simulink model "ParkAssist_Scenario002_cs"  (R2014b)
settings: Solver=ode5  SolverMode=SingleTasking  StartTime=0.0  StopTime=100  FixedStep=1/100  RelTol=1e-3
PreLoadFcn:
  | mbxruntime.callbacks.PreLoadFcn(bdroot);
  | check_NUTS_defined;
  | 
  | assignin('base',['model_closed_' bdroot],false);
  | addpath('../includes_AP');
PostLoadFcn:
  | mbxruntime.callbacks.PostLoadFcn(bdroot);
  | 
  | AP_PlotSpeed;
  | Sim_Stop();
InitFcn:
  | mbxruntime.callbacks.InitFcn(bdroot);
StartFcn:
  | mbxruntime.callbacks.StartFcn(bdroot);
StopFcn:
  | Sim_Stop();
  | 
  | mbxruntime.callbacks.StopFcn(bdroot);
model workspace: external: MAT-File .\ParkAssist_Scenario002_cs_hws.mat (data not in the file)
undefined symbols (not defined in the file or in its folder): mbxruntime, tabledata, warningInitialVelocity, x0
undefined symbols (not defined in the file): ParkAssist_Scenario002_cs_002fddfe84a374e6, ParkAssist_Scenario002_cs_01094a893a7092b9, ParkAssist_Scenario002_cs_02c2e05763b93088, ParkAssist_Scenario002_cs_032149ae54ddfcd1, ParkAssist_Scenario002_cs_03734bce5661314c, ParkAssist_Scenario002_cs_04091ed9282bd749, ParkAssist_Scenario002_cs_068635de1ad515a4, ParkAssist_Scenario002_cs_08968b565ab05e4d, ParkAssist_Scenario002_cs_08eaa26dcd990c9f, ParkAssist_Scenario002_cs_0a721129d3af9f72, ParkAssist_Scenario002_cs_0c5b0314074f54f3, ParkAssist_Scenario002_cs_0e48d515abeb5eec, ParkAssist_Scenario002_cs_1024d8e6ed1cbdcd, ParkAssist_Scenario002_cs_1193d522b107ebab, ParkAssist_Scenario002_cs_11dc16d46c17a7bf, ParkAssist_Scenario002_cs_13631b53806ed88f, ParkAssist_Scenario002_cs_155b57131b5ca1b3, ParkAssist_Scenario002_cs_1a68a29dae7c954c, ParkAssist_Scenario002_cs_1e925263f9fbaeb5, ParkAssist_Scenario002_cs_2102ebaddaee4634, ParkAssist_Scenario002_cs_242d7930853a635b, ParkAssist_Scenario002_cs_26123a651f74a75d, ParkAssist_Scenario002_cs_27077c166553ac4d, ParkAssist_Scenario002_cs_2775446e3f6a532e, ParkAssist_Scenario002_cs_29e1fcc85129d061, ParkAssist_Scenario002_cs_2c6c606bb8eb7e2a, ParkAssist_Scenario002_cs_2f026f6d085d63d4, ParkAssist_Scenario002_cs_2f66cf02f0c1fb02, ParkAssist_Scenario002_cs_2f7abfb8e98983ca, ParkAssist_Scenario002_cs_305144d476c37e1c, ParkAssist_Scenario002_cs_31c4862b0e1d31d2, ParkAssist_Scenario002_cs_3367812933b7aec5, ParkAssist_Scenario002_cs_338ceb4af5dab20a, ParkAssist_Scenario002_cs_359ca59699e4676c, ParkAssist_Scenario002_cs_374ade2de845ad31, ParkAssist_Scenario002_cs_390ab82ad2c54c91, ParkAssist_Scenario002_cs_391805fec31feab6, ParkAssist_Scenario002_cs_3974aed4b8055855, ParkAssist_Scenario002_cs_3a445c73fa984851, ParkAssist_Scenario002_cs_3a54967829cb62c8, ParkAssist_Scenario002_cs_3a60f4e734f7afb5, ParkAssist_Scenario002_cs_3bf2e9c0bde84b70, ParkAssist_Scenario002_cs_3c27f6f01aa99d37, ParkAssist_Scenario002_cs_3cc4b302268f6896, ParkAssist_Scenario002_cs_40419caba47c1546, ParkAssist_Scenario002_cs_42136abd911dac1d, ParkAssist_Scenario002_cs_44b760977392c607, ParkAssist_Scenario002_cs_470135ef0e52cc5f, ParkAssist_Scenario002_cs_48ebb83f5faed864, ParkAssist_Scenario002_cs_4a04bdc7976b10a4, ParkAssist_Scenario002_cs_4b414fc30cdb2355, ParkAssist_Scenario002_cs_4e3c7ad0309ae8ef, ParkAssist_Scenario002_cs_4f1cb442d755f69c, ParkAssist_Scenario002_cs_52f490d0aa621cbf, ParkAssist_Scenario002_cs_53df9d722ee02dea, ParkAssist_Scenario002_cs_5719a2c72af27d7c, ParkAssist_Scenario002_cs_575bfb9c514fb17e, ParkAssist_Scenario002_cs_588d2ca56dde3768, ParkAssist_Scenario002_cs_58ef6c537dd8a6a1, ParkAssist_Scenario002_cs_592f78d63a6470cd ... (+97)
libraries: PreScanUsefulBlocks x57, simulink x55, PreScanSimulinkLibrary x54, simulink_extras x6
(part 9 of 15)

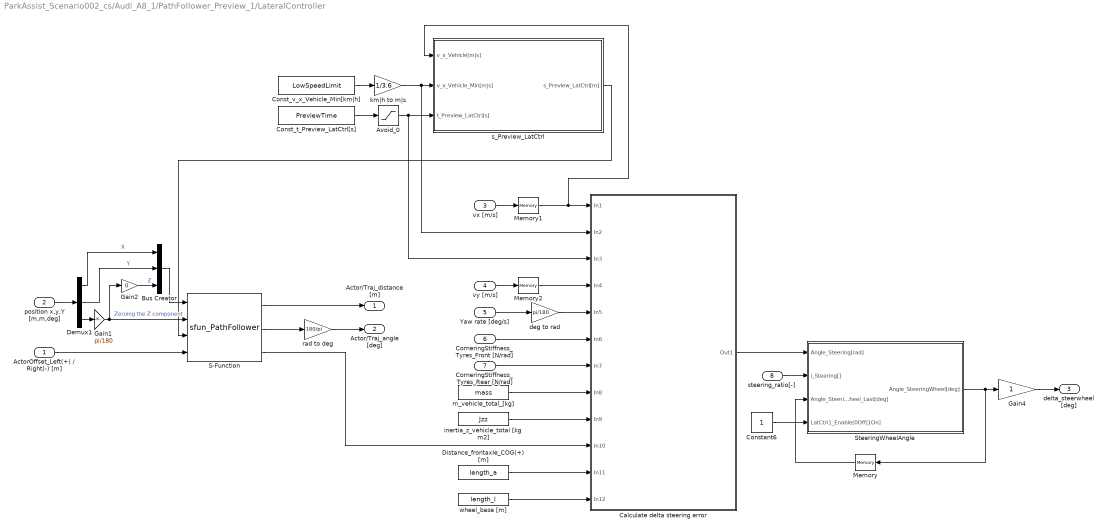
== system ParkAssist_Scenario002_cs/Audi_A8_1/PathFollower_Preview_1/LateralController ==
  ActorOffset_Left(+) / Right(-) [m] : Inport
  position x,y,Y [m,m,deg] : Inport  Port=2
  vx [m/s] : Inport  Port=3
  vy [m/s] : Inport  Port=4
  Yaw rate [deg/s] : Inport  Port=5
  CorneringStiffness_Tyres_Front [N/rad] : Inport  Port=6
  CorneringStiffness_Tyres_Rear [N/rad] : Inport  Port=7
  steering_ratio[-] : Inport  Port=8
  Avoid_0 : Saturate  UpperLimit=1000  LowerLimit=0.1
  Bus Creator : BusCreator  Inputs='X','Y','Z'  OutDataTypeStr=Bus: PRESCAN_XYZ_DATA
  Calculate delta steering error : Subsystem
      mask Display:
      | port_label('input', 1, 'v_x_vehicle [m/s]')
      | port_label('input', 2, 'v_x_vehicle_Min [m/s]')
      | port_label('input', 3, 't_Preview_LatCtrl [s]')
      | port_label('input', 4, 'v_y_vehicle [m/s]')
      | port_label('input', 5, 'yawrate_vehicle [rad/sec]')
      | port_label('input', 6, 'CorneringStiffness_Tyres_Front [N/rad]')
      | port_label('input', 7, 'CorneringStiffness_Tyres_Rear [N/rad]')
      | port_label('input', 8, 'm_vehicle_total [kg]')
      | port_label('input', 9, 'inertia_z_vehicle_total [kg m2]')
      | port_label('input', 10, 'e_Lat [m]')
      | port_label('input', 11, 'Distance_frontaxle_COG(+) [m]')
      | port_label('input', 12, 'wheel_base [m]')
      | port_label('output', 1, 'delta_steeringwheel [rad]')
  Const_t_Preview_LatCtrl[s] : Constant  Value=PreviewTime  SampleTime=CSSampleTime
  Const_v_x_Vehicle_Min[km|h] : Constant  Value=LowSpeedLimit  SampleTime=CSSampleTime
  Constant6 : Constant  SampleTime=CSSampleTime
  Demux1 : Demux  Outputs=3
  Distance_frontaxle_COG(+) [m] : Constant  Value=length_a  SampleTime=CSSampleTime
  Gain1 : Gain  Gain=pi/180
  Gain2 : Gain  Gain=0
  Gain4 : Gain
  Memory : Memory  InheritSampleTime=on
  Memory1 : Memory  InheritSampleTime=on
  Memory2 : Memory  InheritSampleTime=on
  S-Function : S-Function  FunctionName=sfun_PathFollower  Parameters=PathUniqueID,-1  EnableBusSupport=off
  SteeringWheelAngle : Subsystem
  deg to rad : Gain  Gain=pi/180
  inertia_z_vehicle_total [kg m2] : Constant  Value=Jzz  SampleTime=CSSampleTime
  km|h to m|s : Gain  Gain=1/3.6
  m_vehicle_total_[kg] : Constant  Value=mass  SampleTime=CSSampleTime
  rad to deg : Gain  Gain=180/pi
  s_Preview_LatCtrl : Subsystem
  wheel_base [m] : Constant  Value=length_l  SampleTime=CSSampleTime
  Actor/Traj_distance [m] : Outport
  Actor/Traj_angle [deg] : Outport  Port=2
  delta_steerwheel [deg] : Outport  Port=3
  wires:
  Gain2/1 -> Bus Creator/3  "Z"
  Bus Creator/1 -> S-Function/1
  Demux1/2 -> Bus Creator/2  "Y"
  Demux1/1 -> Bus Creator/1  "X"
  s_Preview_LatCtrl/1(s_Preview_LatCtrl[m]) -> S-Function/3
  rad to deg/1 -> Actor/Traj_angle [deg]/1
  km|h to m|s/1 -> Calculate delta steering error/2(In2), s_Preview_LatCtrl/2(v_x_Vehicle_Min[m|s])
  ActorOffset_Left(+) / Right(-) [m]/1 -> S-Function/4
  S-Function/2 -> rad to deg/1
  S-Function/1 -> Actor/Traj_distance [m]/1
  Calculate delta steering error/1(Out1) -> SteeringWheelAngle/1(Angle_Steering[rad])
  vx [m/s]/1 -> Memory1/1
  vy [m/s]/1 -> Memory2/1
  CorneringStiffness_Tyres_Front [N/rad]/1 -> Calculate delta steering error/6(In6)
  m_vehicle_total_[kg]/1 -> Calculate delta steering error/8(In8)
  inertia_z_vehicle_total [kg m2]/1 -> Calculate delta steering error/9(In9)
  steering_ratio[-]/1 -> SteeringWheelAngle/2(i_Steering[])
  SteeringWheelAngle/1(Angle_SteeringWheel[deg]) -> Gain4/1, Memory/1
  Memory/1 -> SteeringWheelAngle/3(Angle_SteeringWheel_Last[deg])
  Constant6/1 -> SteeringWheelAngle/4(LatCtrl1_Enable[0Off|1On])
  Avoid_0/1 -> Calculate delta steering error/3(In3), s_Preview_LatCtrl/3(t_Preview_LatCtrl[s])
  Const_v_x_Vehicle_Min[km|h]/1 -> km|h to m|s/1
  Const_t_Preview_LatCtrl[s]/1 -> Avoid_0/1
  Gain4/1 -> delta_steerwheel [deg]/1
  Distance_frontaxle_COG(+) [m]/1 -> Calculate delta steering error/11(In11)
  CorneringStiffness_Tyres_Rear [N/rad]/1 -> Calculate delta steering error/7(In7)
  Yaw rate [deg/s]/1 -> deg to rad/1
  deg to rad/1 -> Calculate delta steering error/5(In5)
  Gain1/1 -> Gain2/1, S-Function/2  "Zeroing the Z component"
  Demux1/3 -> Gain1/1
  position x,y,Y [m,m,deg]/1 -> Demux1/1
  wheel_base [m]/1 -> Calculate delta steering error/12(In12)
  S-Function/3 -> Calculate delta steering error/10(In10)
  Memory1/1 -> Calculate delta steering error/1(In1), s_Preview_LatCtrl/1(v_x_Vehicle[m|s])
  Memory2/1 -> Calculate delta steering error/4(In4)

== system ParkAssist_Scenario002_cs/Audi_A8_1/PathFollower_Preview_1/LongitudinalController ==
  v_actual [m/s] : Inport
  Desired Velocity [m/s] : Inport  Port=2
  Initial Velocity [m/s] : Inport  Port=3
  Check_Initial_Velocity : Subsystem
  Demux : Demux  Outputs=3
  GearNormal : Constant
  "GearNormal " : Constant
  If Desired Velocity = 0 : Subsystem  TreatAsAtomicUnit=on
  If Desired Velocity ~= 0 : Subsystem  TreatAsAtomicUnit=on
  Memory External IC : Subsystem
  Merge : Merge
  Mux : Mux  Inputs=3
  Mux2 : Mux  Inputs=3
  Sum4 : Sum  Inputs=|+-
  if : If  IfExpression=u1 == 0  SampleTime=CSSampleTime
  throttle [%] : Outport
  brake pressure [bar] : Outport  Port=2
  v0 [m/s] : Outport  Port=3
  Auto_GearShift : Outport  Port=4
  wires:
  v_actual [m/s]/1 -> Check_Initial_Velocity/1(" v_actual_[m|s]"), Memory External IC/1(u)
  Memory External IC/1(y) -> Sum4/2
  Sum4/1 -> If Desired Velocity ~= 0/2(Desired Velocity [m/s])
  Desired Velocity [m/s]/1 -> if/1, Sum4/1
  Initial Velocity [m/s]/1 -> Check_Initial_Velocity/2(Initial_Velocity_[m|s]), Memory External IC/2(IC), v0 [m/s]/1
  GearNormal/1 -> If Desired Velocity = 0/1(In1)
  Merge/1 -> Demux/1
  If Desired Velocity = 0/1(throttle [%]) -> Mux/1
  If Desired Velocity = 0/2(brake pressure [bar]) -> Mux/2
  Mux2/1 -> Merge/2
  Mux/1 -> Merge/1
  Demux/1 -> throttle [%]/1
  Demux/2 -> brake pressure [bar]/1
  Demux/3 -> Auto_GearShift/1
  "GearNormal "/1 -> If Desired Velocity ~= 0/1(In1)
  If Desired Velocity = 0/3(Auto_GearShift) -> Mux/3
  if/2 -> If Desired Velocity ~= 0/Action
  if/1 -> If Desired Velocity = 0/Action
  If Desired Velocity ~= 0/1(throttle [%]) -> Mux2/1
  If Desired Velocity ~= 0/2(brake pressure [bar]) -> Mux2/2
  If Desired Velocity ~= 0/3(Auto_GearShift) -> Mux2/3

== system ParkAssist_Scenario002_cs/Audi_A8_1/SELF_Demux/compas converter ==
  rotz [rad] : Inport
  cart2compas : Subsystem
  rad2deg : Gain  Gain=180/pi
  heading [deg] : Outport
  wires:
  rad2deg/1 -> cart2compas/1(Angle [deg])
  rotz [rad]/1 -> rad2deg/1
  cart2compas/1(heading [deg]) -> heading [deg]/1

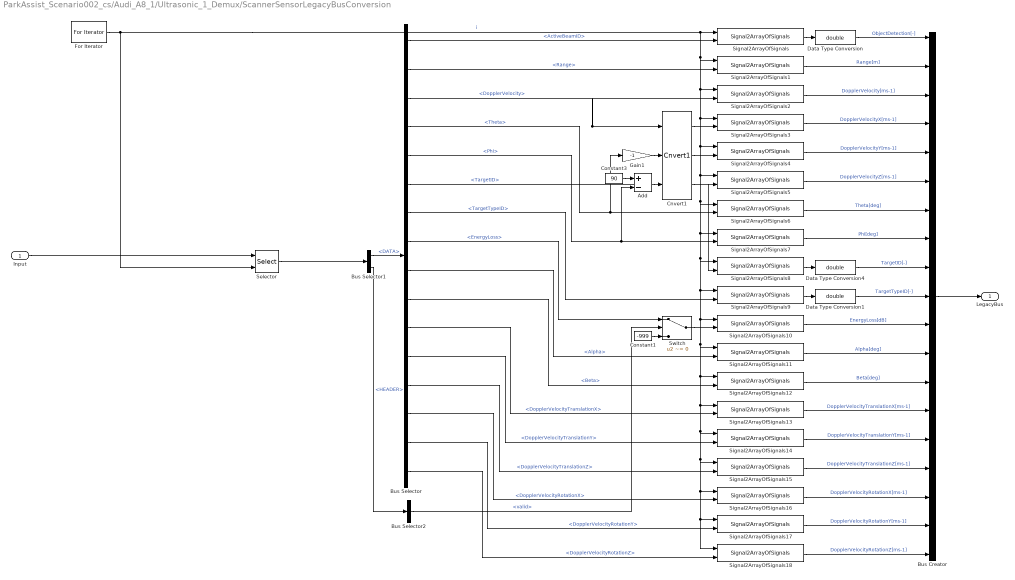
== system ParkAssist_Scenario002_cs/Audi_A8_1/Ultrasonic_1_Demux/ScannerSensorLegacyBusConversion ==
  Input : Inport
  Add : Sum  Inputs=+-
  Bus Creator : BusCreator  Inputs=19
  Bus Selector : BusSelector  OutputSignals=ActiveBeamID,Range,DopplerVelocity,Theta,Phi,TargetID,TargetTypeID,EnergyLoss,Alpha,Beta,DopplerVelocityTranslationX,DopplerVelocityTranslationY,DopplerVelocityTranslationZ,DopplerVelocityRotationX,DopplerVelocityRotationY,DopplerVelocityRotationZ
  Bus Selector1 : BusSelector  OutputSignals=DATA,HEADER
  Bus Selector2 : BusSelector  OutputSignals=valid
  Cnvert1 : PreScanSimulinkLibrary/Cnvert1
  Constant1 : Constant  Value=-999
  Constant3 : Constant  Value=90
  Data Type Conversion : DataTypeConversion  OutDataTypeStr=double  LockScale=on
  Data Type Conversion1 : DataTypeConversion  OutDataTypeStr=double  LockScale=on
  Data Type Conversion4 : DataTypeConversion  OutDataTypeStr=double  LockScale=on
  For Iterator : ForIterator  ResetStates=reset  IterationLimit=MAXMESSAGES
  Gain1 : Gain  Gain=-1
  Selector : Selector  InputPortWidth=MAXMESSAGES  IndexOptions=Index vector (port)  Indices=[1 3]
  Signal2ArrayOfSignals{,1..18} (19 alike) : PreScanUsefulBlocks/Signal2ArrayOfSignals  VECTORLENGTH=MAXMESSAGES
  Switch : Switch  Criteria=u2 ~= 0  Threshold=1
  LegacyBus : Outport
  wires:
  Bus Creator/1 -> LegacyBus/1
  Signal2ArrayOfSignals12/1 -> Bus Creator/13  "Beta[deg]"
  Signal2ArrayOfSignals11/1 -> Bus Creator/12  "Alpha[deg]"
  Signal2ArrayOfSignals10/1 -> Bus Creator/11  "EnergyLoss[dB]"
  Data Type Conversion1/1 -> Bus Creator/10  "TargetTypeID[-]"
  Data Type Conversion4/1 -> Bus Creator/9  "TargetID[-]"
  Signal2ArrayOfSignals7/1 -> Bus Creator/8  "Phi[deg]"
  Signal2ArrayOfSignals6/1 -> Bus Creator/7  "Theta[deg]"
  Signal2ArrayOfSignals5/1 -> Bus Creator/6  "DopplerVelocityZ[ms-1]"
  Signal2ArrayOfSignals4/1 -> Bus Creator/5  "DopplerVelocityY[ms-1]"
  Signal2ArrayOfSignals3/1 -> Bus Creator/4  "DopplerVelocityX[ms-1]"
  Signal2ArrayOfSignals2/1 -> Bus Creator/3  "DopplerVelocity[ms-1]"
  Signal2ArrayOfSignals1/1 -> Bus Creator/2  "Range[m]"
  Data Type Conversion/1 -> Bus Creator/1  "ObjectDetection[-]"
  Signal2ArrayOfSignals9/1 -> Data Type Conversion1/1
  Bus Selector2/1 -> Switch/2  "<valid>"
  Bus Selector1/2 -> Bus Selector2/1  "<HEADER>"
  Bus Selector1/1 -> Bus Selector/1  "<DATA>"
  Switch/1 -> Signal2ArrayOfSignals10/2
  Constant1/1 -> Switch/3
  Bus Selector/8 -> Switch/1  "<EnergyLoss>"
  Selector/1 -> Bus Selector1/1
  Constant3/1 -> Add/1
  Add/1 -> Cnvert1/3
  Gain1/1 -> Cnvert1/2
  Cnvert1/3 -> Signal2ArrayOfSignals5/2
  Cnvert1/2 -> Signal2ArrayOfSignals4/2
  Cnvert1/1 -> Signal2ArrayOfSignals3/2
  Signal2ArrayOfSignals8/1 -> Data Type Conversion4/1
  Bus Selector/1 -> Signal2ArrayOfSignals/2  "<ActiveBeamID>"
  Bus Selector/2 -> Signal2ArrayOfSignals1/2  "<Range>"
  Bus Selector/3 -> Signal2ArrayOfSignals2/2, Cnvert1/1  "<DopplerVelocity>"
  Bus Selector/4 -> Signal2ArrayOfSignals6/2, Gain1/1  "<Theta>"
  Bus Selector/5 -> Signal2ArrayOfSignals7/2, Add/2  "<Phi>"
  Bus Selector/6 -> Signal2ArrayOfSignals8/2  "<TargetID>"
  Bus Selector/7 -> Signal2ArrayOfSignals9/2  "<TargetTypeID>"
  Bus Selector/9 -> Signal2ArrayOfSignals11/2  "<Alpha>"
  Bus Selector/10 -> Signal2ArrayOfSignals12/2  "<Beta>"
  Signal2ArrayOfSignals/1 -> Data Type Conversion/1
  For Iterator/1 -> Signal2ArrayOfSignals11/1, Signal2ArrayOfSignals12/1, Signal2ArrayOfSignals13/1, Signal2ArrayOfSignals14/1, Signal2ArrayOfSignals15/1, Signal2ArrayOfSignals16/1, Signal2ArrayOfSignals17/1, Signal2ArrayOfSignals18/1, Signal2ArrayOfSignals10/1, Signal2ArrayOfSignals9/1, Signal2ArrayOfSignals8/1, Signal2ArrayOfSignals7/1, Signal2ArrayOfSignals6/1, Signal2ArrayOfSignals5/1, Signal2ArrayOfSignals4/1, Signal2ArrayOfSignals3/1, Signal2ArrayOfSignals2/1, Signal2ArrayOfSignals1/1, Signal2ArrayOfSignals/1, Selector/2  "i"
  Input/1 -> Selector/1
  Bus Selector/11 -> Signal2ArrayOfSignals13/2  "<DopplerVelocityTranslationX>"
  Bus Selector/12 -> Signal2ArrayOfSignals14/2  "<DopplerVelocityTranslationY>"
  Bus Selector/13 -> Signal2ArrayOfSignals15/2  "<DopplerVelocityTranslationZ>"
  Bus Selector/14 -> Signal2ArrayOfSignals16/2  "<DopplerVelocityRotationX>"
  Bus Selector/15 -> Signal2ArrayOfSignals17/2  "<DopplerVelocityRotationY>"
  Bus Selector/16 -> Signal2ArrayOfSignals18/2  "<DopplerVelocityRotationZ>"
  Signal2ArrayOfSignals13/1 -> Bus Creator/14  "DopplerVelocityTranslationX[ms-1]"
  Signal2ArrayOfSignals14/1 -> Bus Creator/15  "DopplerVelocityTranslationY[ms-1]"
  Signal2ArrayOfSignals15/1 -> Bus Creator/16  "DopplerVelocityTranslationZ[ms-1]"
  Signal2ArrayOfSignals16/1 -> Bus Creator/17  "DopplerVelocityRotationX[ms-1]"
  Signal2ArrayOfSignals17/1 -> Bus Creator/18  "DopplerVelocityRotationY[ms-1]"
  Signal2ArrayOfSignals18/1 -> Bus Creator/19  "DopplerVelocityRotationZ[ms-1]"

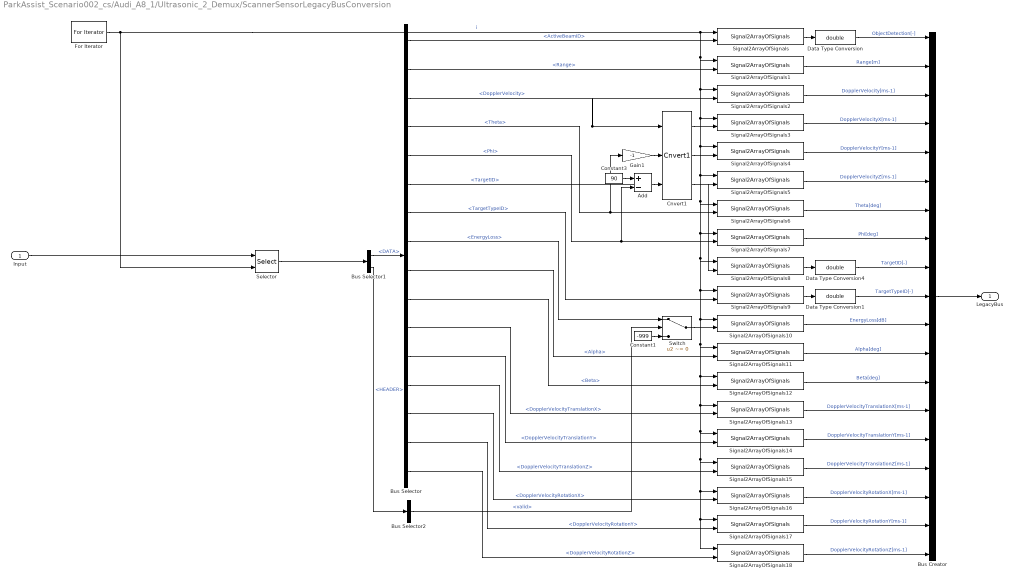
== system ParkAssist_Scenario002_cs/Audi_A8_1/Ultrasonic_2_Demux/ScannerSensorLegacyBusConversion ==
  Input : Inport
  Add : Sum  Inputs=+-
  Bus Creator : BusCreator  Inputs=19
  Bus Selector : BusSelector  OutputSignals=ActiveBeamID,Range,DopplerVelocity,Theta,Phi,TargetID,TargetTypeID,EnergyLoss,Alpha,Beta,DopplerVelocityTranslationX,DopplerVelocityTranslationY,DopplerVelocityTranslationZ,DopplerVelocityRotationX,DopplerVelocityRotationY,DopplerVelocityRotationZ
  Bus Selector1 : BusSelector  OutputSignals=DATA,HEADER
  Bus Selector2 : BusSelector  OutputSignals=valid
  Cnvert1 : PreScanSimulinkLibrary/Cnvert1
  Constant1 : Constant  Value=-999
  Constant3 : Constant  Value=90
  Data Type Conversion : DataTypeConversion  OutDataTypeStr=double  LockScale=on
  Data Type Conversion1 : DataTypeConversion  OutDataTypeStr=double  LockScale=on
  Data Type Conversion4 : DataTypeConversion  OutDataTypeStr=double  LockScale=on
  For Iterator : ForIterator  ResetStates=reset  IterationLimit=MAXMESSAGES
  Gain1 : Gain  Gain=-1
  Selector : Selector  InputPortWidth=MAXMESSAGES  IndexOptions=Index vector (port)  Indices=[1 3]
  Signal2ArrayOfSignals{,1..18} (19 alike) : PreScanUsefulBlocks/Signal2ArrayOfSignals  VECTORLENGTH=MAXMESSAGES
  Switch : Switch  Criteria=u2 ~= 0  Threshold=1
  LegacyBus : Outport
  wires:
  Bus Creator/1 -> LegacyBus/1
  Signal2ArrayOfSignals12/1 -> Bus Creator/13  "Beta[deg]"
  Signal2ArrayOfSignals11/1 -> Bus Creator/12  "Alpha[deg]"
  Signal2ArrayOfSignals10/1 -> Bus Creator/11  "EnergyLoss[dB]"
  Data Type Conversion1/1 -> Bus Creator/10  "TargetTypeID[-]"
  Data Type Conversion4/1 -> Bus Creator/9  "TargetID[-]"
  Signal2ArrayOfSignals7/1 -> Bus Creator/8  "Phi[deg]"
  Signal2ArrayOfSignals6/1 -> Bus Creator/7  "Theta[deg]"
  Signal2ArrayOfSignals5/1 -> Bus Creator/6  "DopplerVelocityZ[ms-1]"
  Signal2ArrayOfSignals4/1 -> Bus Creator/5  "DopplerVelocityY[ms-1]"
  Signal2ArrayOfSignals3/1 -> Bus Creator/4  "DopplerVelocityX[ms-1]"
  Signal2ArrayOfSignals2/1 -> Bus Creator/3  "DopplerVelocity[ms-1]"
  Signal2ArrayOfSignals1/1 -> Bus Creator/2  "Range[m]"
  Data Type Conversion/1 -> Bus Creator/1  "ObjectDetection[-]"
  Signal2ArrayOfSignals9/1 -> Data Type Conversion1/1
  Bus Selector2/1 -> Switch/2  "<valid>"
  Bus Selector1/2 -> Bus Selector2/1  "<HEADER>"
  Bus Selector1/1 -> Bus Selector/1  "<DATA>"
  Switch/1 -> Signal2ArrayOfSignals10/2
  Constant1/1 -> Switch/3
  Bus Selector/8 -> Switch/1  "<EnergyLoss>"
  Selector/1 -> Bus Selector1/1
  Constant3/1 -> Add/1
  Add/1 -> Cnvert1/3
  Gain1/1 -> Cnvert1/2
  Cnvert1/3 -> Signal2ArrayOfSignals5/2
  Cnvert1/2 -> Signal2ArrayOfSignals4/2
  Cnvert1/1 -> Signal2ArrayOfSignals3/2
  Signal2ArrayOfSignals8/1 -> Data Type Conversion4/1
  Bus Selector/1 -> Signal2ArrayOfSignals/2  "<ActiveBeamID>"
  Bus Selector/2 -> Signal2ArrayOfSignals1/2  "<Range>"
  Bus Selector/3 -> Signal2ArrayOfSignals2/2, Cnvert1/1  "<DopplerVelocity>"
  Bus Selector/4 -> Signal2ArrayOfSignals6/2, Gain1/1  "<Theta>"
  Bus Selector/5 -> Signal2ArrayOfSignals7/2, Add/2  "<Phi>"
  Bus Selector/6 -> Signal2ArrayOfSignals8/2  "<TargetID>"
  Bus Selector/7 -> Signal2ArrayOfSignals9/2  "<TargetTypeID>"
  Bus Selector/9 -> Signal2ArrayOfSignals11/2  "<Alpha>"
  Bus Selector/10 -> Signal2ArrayOfSignals12/2  "<Beta>"
  Signal2ArrayOfSignals/1 -> Data Type Conversion/1
  For Iterator/1 -> Signal2ArrayOfSignals11/1, Signal2ArrayOfSignals12/1, Signal2ArrayOfSignals13/1, Signal2ArrayOfSignals14/1, Signal2ArrayOfSignals15/1, Signal2ArrayOfSignals16/1, Signal2ArrayOfSignals17/1, Signal2ArrayOfSignals18/1, Signal2ArrayOfSignals10/1, Signal2ArrayOfSignals9/1, Signal2ArrayOfSignals8/1, Signal2ArrayOfSignals7/1, Signal2ArrayOfSignals6/1, Signal2ArrayOfSignals5/1, Signal2ArrayOfSignals4/1, Signal2ArrayOfSignals3/1, Signal2ArrayOfSignals2/1, Signal2ArrayOfSignals1/1, Signal2ArrayOfSignals/1, Selector/2  "i"
  Input/1 -> Selector/1
  Bus Selector/11 -> Signal2ArrayOfSignals13/2  "<DopplerVelocityTranslationX>"
  Bus Selector/12 -> Signal2ArrayOfSignals14/2  "<DopplerVelocityTranslationY>"
  Bus Selector/13 -> Signal2ArrayOfSignals15/2  "<DopplerVelocityTranslationZ>"
  Bus Selector/14 -> Signal2ArrayOfSignals16/2  "<DopplerVelocityRotationX>"
  Bus Selector/15 -> Signal2ArrayOfSignals17/2  "<DopplerVelocityRotationY>"
  Bus Selector/16 -> Signal2ArrayOfSignals18/2  "<DopplerVelocityRotationZ>"
  Signal2ArrayOfSignals13/1 -> Bus Creator/14  "DopplerVelocityTranslationX[ms-1]"
  Signal2ArrayOfSignals14/1 -> Bus Creator/15  "DopplerVelocityTranslationY[ms-1]"
  Signal2ArrayOfSignals15/1 -> Bus Creator/16  "DopplerVelocityTranslationZ[ms-1]"
  Signal2ArrayOfSignals16/1 -> Bus Creator/17  "DopplerVelocityRotationX[ms-1]"
  Signal2ArrayOfSignals17/1 -> Bus Creator/18  "DopplerVelocityRotationY[ms-1]"
  Signal2ArrayOfSignals18/1 -> Bus Creator/19  "DopplerVelocityRotationZ[ms-1]"

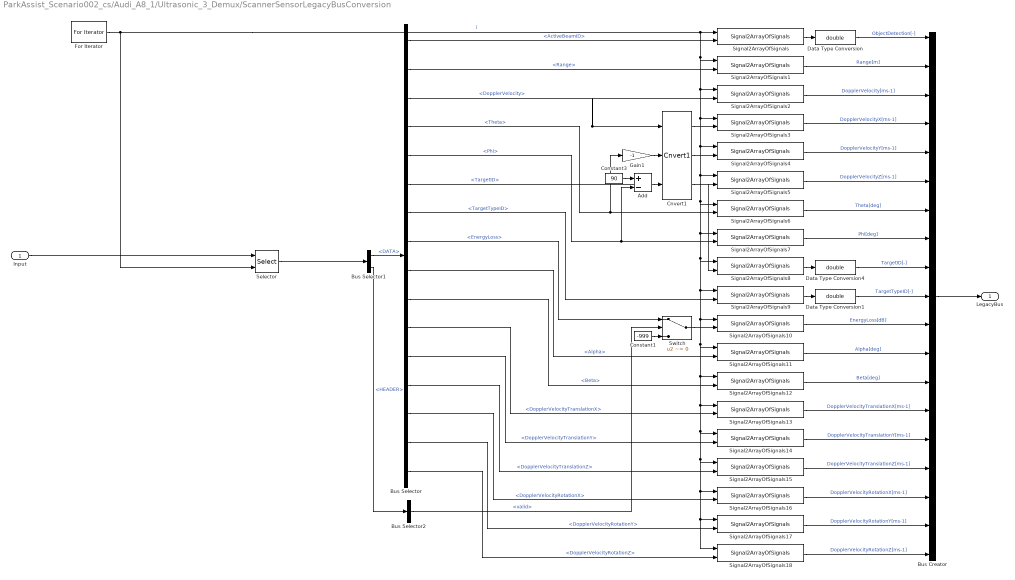
== system ParkAssist_Scenario002_cs/Audi_A8_1/Ultrasonic_3_Demux/ScannerSensorLegacyBusConversion ==
  Input : Inport
  Add : Sum  Inputs=+-
  Bus Creator : BusCreator  Inputs=19
  Bus Selector : BusSelector  OutputSignals=ActiveBeamID,Range,DopplerVelocity,Theta,Phi,TargetID,TargetTypeID,EnergyLoss,Alpha,Beta,DopplerVelocityTranslationX,DopplerVelocityTranslationY,DopplerVelocityTranslationZ,DopplerVelocityRotationX,DopplerVelocityRotationY,DopplerVelocityRotationZ
  Bus Selector1 : BusSelector  OutputSignals=DATA,HEADER
  Bus Selector2 : BusSelector  OutputSignals=valid
  Cnvert1 : PreScanSimulinkLibrary/Cnvert1
  Constant1 : Constant  Value=-999
  Constant3 : Constant  Value=90
  Data Type Conversion : DataTypeConversion  OutDataTypeStr=double  LockScale=on
  Data Type Conversion1 : DataTypeConversion  OutDataTypeStr=double  LockScale=on
  Data Type Conversion4 : DataTypeConversion  OutDataTypeStr=double  LockScale=on
  For Iterator : ForIterator  ResetStates=reset  IterationLimit=MAXMESSAGES
  Gain1 : Gain  Gain=-1
  Selector : Selector  InputPortWidth=MAXMESSAGES  IndexOptions=Index vector (port)  Indices=[1 3]
  Signal2ArrayOfSignals{,1..18} (19 alike) : PreScanUsefulBlocks/Signal2ArrayOfSignals  VECTORLENGTH=MAXMESSAGES
  Switch : Switch  Criteria=u2 ~= 0  Threshold=1
  LegacyBus : Outport
  wires:
  Bus Creator/1 -> LegacyBus/1
  Signal2ArrayOfSignals12/1 -> Bus Creator/13  "Beta[deg]"
  Signal2ArrayOfSignals11/1 -> Bus Creator/12  "Alpha[deg]"
  Signal2ArrayOfSignals10/1 -> Bus Creator/11  "EnergyLoss[dB]"
  Data Type Conversion1/1 -> Bus Creator/10  "TargetTypeID[-]"
  Data Type Conversion4/1 -> Bus Creator/9  "TargetID[-]"
  Signal2ArrayOfSignals7/1 -> Bus Creator/8  "Phi[deg]"
  Signal2ArrayOfSignals6/1 -> Bus Creator/7  "Theta[deg]"
  Signal2ArrayOfSignals5/1 -> Bus Creator/6  "DopplerVelocityZ[ms-1]"
  Signal2ArrayOfSignals4/1 -> Bus Creator/5  "DopplerVelocityY[ms-1]"
  Signal2ArrayOfSignals3/1 -> Bus Creator/4  "DopplerVelocityX[ms-1]"
  Signal2ArrayOfSignals2/1 -> Bus Creator/3  "DopplerVelocity[ms-1]"
  Signal2ArrayOfSignals1/1 -> Bus Creator/2  "Range[m]"
  Data Type Conversion/1 -> Bus Creator/1  "ObjectDetection[-]"
  Signal2ArrayOfSignals9/1 -> Data Type Conversion1/1
  Bus Selector2/1 -> Switch/2  "<valid>"
  Bus Selector1/2 -> Bus Selector2/1  "<HEADER>"
  Bus Selector1/1 -> Bus Selector/1  "<DATA>"
  Switch/1 -> Signal2ArrayOfSignals10/2
  Constant1/1 -> Switch/3
  Bus Selector/8 -> Switch/1  "<EnergyLoss>"
  Selector/1 -> Bus Selector1/1
  Constant3/1 -> Add/1
  Add/1 -> Cnvert1/3
  Gain1/1 -> Cnvert1/2
  Cnvert1/3 -> Signal2ArrayOfSignals5/2
  Cnvert1/2 -> Signal2ArrayOfSignals4/2
  Cnvert1/1 -> Signal2ArrayOfSignals3/2
  Signal2ArrayOfSignals8/1 -> Data Type Conversion4/1
  Bus Selector/1 -> Signal2ArrayOfSignals/2  "<ActiveBeamID>"
  Bus Selector/2 -> Signal2ArrayOfSignals1/2  "<Range>"
  Bus Selector/3 -> Signal2ArrayOfSignals2/2, Cnvert1/1  "<DopplerVelocity>"
  Bus Selector/4 -> Signal2ArrayOfSignals6/2, Gain1/1  "<Theta>"
  Bus Selector/5 -> Signal2ArrayOfSignals7/2, Add/2  "<Phi>"
  Bus Selector/6 -> Signal2ArrayOfSignals8/2  "<TargetID>"
  Bus Selector/7 -> Signal2ArrayOfSignals9/2  "<TargetTypeID>"
  Bus Selector/9 -> Signal2ArrayOfSignals11/2  "<Alpha>"
  Bus Selector/10 -> Signal2ArrayOfSignals12/2  "<Beta>"
  Signal2ArrayOfSignals/1 -> Data Type Conversion/1
  For Iterator/1 -> Signal2ArrayOfSignals11/1, Signal2ArrayOfSignals12/1, Signal2ArrayOfSignals13/1, Signal2ArrayOfSignals14/1, Signal2ArrayOfSignals15/1, Signal2ArrayOfSignals16/1, Signal2ArrayOfSignals17/1, Signal2ArrayOfSignals18/1, Signal2ArrayOfSignals10/1, Signal2ArrayOfSignals9/1, Signal2ArrayOfSignals8/1, Signal2ArrayOfSignals7/1, Signal2ArrayOfSignals6/1, Signal2ArrayOfSignals5/1, Signal2ArrayOfSignals4/1, Signal2ArrayOfSignals3/1, Signal2ArrayOfSignals2/1, Signal2ArrayOfSignals1/1, Signal2ArrayOfSignals/1, Selector/2  "i"
  Input/1 -> Selector/1
  Bus Selector/11 -> Signal2ArrayOfSignals13/2  "<DopplerVelocityTranslationX>"
  Bus Selector/12 -> Signal2ArrayOfSignals14/2  "<DopplerVelocityTranslationY>"
  Bus Selector/13 -> Signal2ArrayOfSignals15/2  "<DopplerVelocityTranslationZ>"
  Bus Selector/14 -> Signal2ArrayOfSignals16/2  "<DopplerVelocityRotationX>"
  Bus Selector/15 -> Signal2ArrayOfSignals17/2  "<DopplerVelocityRotationY>"
  Bus Selector/16 -> Signal2ArrayOfSignals18/2  "<DopplerVelocityRotationZ>"
  Signal2ArrayOfSignals13/1 -> Bus Creator/14  "DopplerVelocityTranslationX[ms-1]"
  Signal2ArrayOfSignals14/1 -> Bus Creator/15  "DopplerVelocityTranslationY[ms-1]"
  Signal2ArrayOfSignals15/1 -> Bus Creator/16  "DopplerVelocityTranslationZ[ms-1]"
  Signal2ArrayOfSignals16/1 -> Bus Creator/17  "DopplerVelocityRotationX[ms-1]"
  Signal2ArrayOfSignals17/1 -> Bus Creator/18  "DopplerVelocityRotationY[ms-1]"
  Signal2ArrayOfSignals18/1 -> Bus Creator/19  "DopplerVelocityRotationZ[ms-1]"

== system ParkAssist_Scenario002_cs/Audi_A8_1/WheelDisplacement_Mux/WheelL0_Mux ==
  X [m] : Inport
  Y [m] : Inport  Port=2
  Z [m] : Inport  Port=3
  Roll [rad] : Inport  Port=4
  Pitch [rad] : Inport  Port=5
  Yaw [rad] : Inport  Port=6
  Bus Creator : BusCreator  Inputs=3  OutDataTypeStr=Bus: PRESCAN_XYZ_DATA
  Bus Creator1 : BusCreator  Inputs=3  OutDataTypeStr=Bus: PRESCAN_RPY_DATA
  Bus Creator2 : BusCreator  Inputs=2  OutDataTypeStr=Bus: PRESCAN_POSE_DATA
  Joint : Outport
  wires:
  Yaw [rad]/1 -> Bus Creator1/3  "Yaw"
  Bus Creator1/1 -> Bus Creator2/2  "ORIENTATION"
  Bus Creator/1 -> Bus Creator2/1  "POSITION"
  X [m]/1 -> Bus Creator/1  "X"
  Y [m]/1 -> Bus Creator/2  "Y"
  Z [m]/1 -> Bus Creator/3  "Z"
  Bus Creator2/1 -> Joint/1
  Roll [rad]/1 -> Bus Creator1/1  "Roll"
  Pitch [rad]/1 -> Bus Creator1/2  "Pitch"

== system ParkAssist_Scenario002_cs/Audi_A8_1/WheelDisplacement_Mux/WheelL1_Mux ==
  X [m] : Inport
  Y [m] : Inport  Port=2
  Z [m] : Inport  Port=3
  Roll [rad] : Inport  Port=4
  Pitch [rad] : Inport  Port=5
  Yaw [rad] : Inport  Port=6
  Bus Creator : BusCreator  Inputs=3  OutDataTypeStr=Bus: PRESCAN_XYZ_DATA
  Bus Creator1 : BusCreator  Inputs=3  OutDataTypeStr=Bus: PRESCAN_RPY_DATA
  Bus Creator2 : BusCreator  Inputs=2  OutDataTypeStr=Bus: PRESCAN_POSE_DATA
  Joint : Outport
  wires:
  Yaw [rad]/1 -> Bus Creator1/3  "Yaw"
  Bus Creator1/1 -> Bus Creator2/2  "ORIENTATION"
  Bus Creator/1 -> Bus Creator2/1  "POSITION"
  X [m]/1 -> Bus Creator/1  "X"
  Y [m]/1 -> Bus Creator/2  "Y"
  Z [m]/1 -> Bus Creator/3  "Z"
  Bus Creator2/1 -> Joint/1
  Roll [rad]/1 -> Bus Creator1/1  "Roll"
  Pitch [rad]/1 -> Bus Creator1/2  "Pitch"

== system ParkAssist_Scenario002_cs/Audi_A8_1/WheelDisplacement_Mux/WheelR0_Mux ==
  X [m] : Inport
  Y [m] : Inport  Port=2
  Z [m] : Inport  Port=3
  Roll [rad] : Inport  Port=4
  Pitch [rad] : Inport  Port=5
  Yaw [rad] : Inport  Port=6
  Bus Creator : BusCreator  Inputs=3  OutDataTypeStr=Bus: PRESCAN_XYZ_DATA
  Bus Creator1 : BusCreator  Inputs=3  OutDataTypeStr=Bus: PRESCAN_RPY_DATA
  Bus Creator2 : BusCreator  Inputs=2  OutDataTypeStr=Bus: PRESCAN_POSE_DATA
  Joint : Outport
  wires:
  Yaw [rad]/1 -> Bus Creator1/3  "Yaw"
  Bus Creator1/1 -> Bus Creator2/2  "ORIENTATION"
  Bus Creator/1 -> Bus Creator2/1  "POSITION"
  X [m]/1 -> Bus Creator/1  "X"
  Y [m]/1 -> Bus Creator/2  "Y"
  Z [m]/1 -> Bus Creator/3  "Z"
  Bus Creator2/1 -> Joint/1
  Roll [rad]/1 -> Bus Creator1/1  "Roll"
  Pitch [rad]/1 -> Bus Creator1/2  "Pitch"

== system ParkAssist_Scenario002_cs/Audi_A8_1/WheelDisplacement_Mux/WheelR1_Mux ==
  X [m] : Inport
  Y [m] : Inport  Port=2
  Z [m] : Inport  Port=3
  Roll [rad] : Inport  Port=4
  Pitch [rad] : Inport  Port=5
  Yaw [rad] : Inport  Port=6
  Bus Creator : BusCreator  Inputs=3  OutDataTypeStr=Bus: PRESCAN_XYZ_DATA
  Bus Creator1 : BusCreator  Inputs=3  OutDataTypeStr=Bus: PRESCAN_RPY_DATA
  Bus Creator2 : BusCreator  Inputs=2  OutDataTypeStr=Bus: PRESCAN_POSE_DATA
  Joint : Outport
  wires:
  Yaw [rad]/1 -> Bus Creator1/3  "Yaw"
  Bus Creator1/1 -> Bus Creator2/2  "ORIENTATION"
  Bus Creator/1 -> Bus Creator2/1  "POSITION"
  X [m]/1 -> Bus Creator/1  "X"
  Y [m]/1 -> Bus Creator/2  "Y"
  Z [m]/1 -> Bus Creator/3  "Z"
  Bus Creator2/1 -> Joint/1
  Roll [rad]/1 -> Bus Creator1/1  "Roll"
  Pitch [rad]/1 -> Bus Creator1/2  "Pitch"

== system ParkAssist_Scenario002_cs/Audi_A8_10/Dynamics_Empty/MuxState ==
  note: mode: Dynamics
  note: mode: Positioning
  note: mode: Dynamics
      | VelVEHICLE
      | wrt VEH
  note: AnglesVEHICLE
      | wrtGLOB
  note: For state mode 'Dynamic' positions
      | are not taken into account, as they
      | are computed by integrating velocity.
      | Click annotation for Help.
  x [m] : Inport  SampleTime=TimeStep
  y [m] : Inport  Port=2  SampleTime=TimeStep
  z [m] : Inport  Port=3  SampleTime=TimeStep
  dx [m/s] : Inport  Port=4  SampleTime=TimeStep
  dy [m/s] : Inport  Port=5  SampleTime=TimeStep
  dz [m/s] : Inport  Port=6  SampleTime=TimeStep
  R [rad] : Inport  Port=7  SampleTime=TimeStep
  P [rad] : Inport  Port=8  SampleTime=TimeStep
  Y [rad] : Inport  Port=9  SampleTime=TimeStep
  Constant : Constant  DisableCoverage=on  Value=positioningmode
  Discrete-Time Integrator : DiscreteIntegrator  SampleTime=TimeStep
  Ground : Ground
  Ground1 : Ground
  Mux1 : Mux  Inputs=[3 3]
  Mux2 : Mux  Inputs=3
  Mux3 : Mux  Inputs=3
  Mux4 : Mux  Inputs=3
  Mux5 : Mux  Inputs=[3 3]
  Mux6 : Mux  Inputs=[6 3]
  Switch : Switch  Threshold=0.5
  Transformation_BODY2GLOBAL : PreScanSimulinkLibrary/Simple_Vehicle_Dynamics/Chassis/MuxDynState/Transformation_BODY2GLOBAL
  mux3 : Mux  Inputs=3
  state : Outport
  wires:
  Constant/1 -> Switch/2
  Mux6/1 -> state/1
  Mux4/1 -> Mux1/1
  Mux5/1 -> Switch/3
  Mux1/1 -> Switch/1
  Switch/1 -> Mux6/1  "PosVeh wrt  GLOB"
  P [rad]/1 -> Mux3/2
  R [rad]/1 -> Mux3/1
  dz [m/s]/1 -> Mux2/3
  dy [m/s]/1 -> Mux2/2
  dx [m/s]/1 -> Mux2/1
  z [m]/1 -> Mux4/3
  y [m]/1 -> Mux4/2
  x [m]/1 -> Mux4/1
  Ground1/1 -> mux3/2  "pitch"
  Y [rad]/1 -> mux3/3, Mux3/3  "yaw"
  Mux3/1 -> Mux6/2
  Transformation_BODY2GLOBAL/1 -> Discrete-Time Integrator/1, Mux5/2  "VelVEH wrt  GLOB"
  mux3/1 -> Transformation_BODY2GLOBAL/2
  Ground/1 -> mux3/1  "roll"
  Mux2/1 -> Mux1/2, Transformation_BODY2GLOBAL/1
  Discrete-Time Integrator/1 -> Mux5/1  "PosVEH wrt  GLOB"

== system ParkAssist_Scenario002_cs/Audi_A8_10/Dynamics_Empty/STATE_Audi_A8_10 ==
  State : Inport  SampleTime=TimeStep
  Bus Creator : BusCreator  Inputs=15  OutDataTypeStr=Bus: PRESCAN_STATEACTUATORDATA  NonVirtualBus=on
  Constant : Constant  Value=0
  Demux : Demux  Outputs=15
  Mux : Mux  Inputs=3
  Mux1 : Mux  Inputs=3
  Mux2 : Mux  Inputs=3
  iniBODYAngles wrtVEH [rad] : Constant  Value=Roll0  SampleTime=TimeStep
  iniBODYAngles wrtVEH [rad]1 : Constant  Value=Pitch0  SampleTime=TimeStep
  iniVEHAngles wrtGLOB [rad] : Constant  Value=Yaw0  SampleTime=TimeStep
  iniVEHposition wrtGLOB [m] : Constant  Value=x0  SampleTime=TimeStep
  iniVEHposition wrtGLOB [m]1 : Constant  Value=y0  SampleTime=TimeStep
  iniVEHposition wrtGLOB [m]2 : Constant  Value=z0  SampleTime=TimeStep
  state2FullState : PreScanSimulinkLibrary/state2FullState  SystemSampleTime=-1
  StateBus : Outport  OutDataTypeStr=Bus: PRESCAN_STATEACTUATORDATA
  wires:
  Mux2/1 -> state2FullState/4
  iniVEHAngles wrtGLOB [rad]/1 -> Mux2/3
  Mux1/1 -> state2FullState/3
  Constant/1 -> Mux2/1, Mux2/2, Mux1/3
  iniBODYAngles wrtVEH [rad]1/1 -> Mux1/2
  iniBODYAngles wrtVEH [rad]/1 -> Mux1/1
  Mux/1 -> state2FullState/2
  iniVEHposition wrtGLOB [m]2/1 -> Mux/3
  iniVEHposition wrtGLOB [m]/1 -> Mux/1
  iniVEHposition wrtGLOB [m]1/1 -> Mux/2
  Demux/15 -> Bus Creator/15  "AngularVelocityYaw"
  Demux/14 -> Bus Creator/14  "AngularVelocityPitch"
  Demux/13 -> Bus Creator/13  "AngularVelocityRoll"
  Demux/12 -> Bus Creator/12  "OrientationYaw"
  Demux/11 -> Bus Creator/11  "OrientationPitch"
  Demux/10 -> Bus Creator/10  "OrientationRoll"
  Demux/9 -> Bus Creator/9  "AccelerationZ"
  Demux/8 -> Bus Creator/8  "AccelerationY"
  Demux/7 -> Bus Creator/7  "AccelerationX"
  Demux/6 -> Bus Creator/6  "VelocityZ"
  Demux/5 -> Bus Creator/5  "VelocityY"
  Demux/4 -> Bus Creator/4  "VelocityX"
  Demux/3 -> Bus Creator/3  "PositionZ"
  Demux/2 -> Bus Creator/2  "PositionY"
  Demux/1 -> Bus Creator/1  "PositionX"
  state2FullState/1 -> Demux/1
  State/1 -> state2FullState/1
  Bus Creator/1 -> StateBus/1

== system ParkAssist_Scenario002_cs/Audi_A8_10/SELF_Demux/compas converter ==
  rotz [rad] : Inport
  cart2compas : Subsystem
  rad2deg : Gain  Gain=180/pi
  heading [deg] : Outport
  wires:
  rad2deg/1 -> cart2compas/1(Angle [deg])
  rotz [rad]/1 -> rad2deg/1
  cart2compas/1(heading [deg]) -> heading [deg]/1

== system ParkAssist_Scenario002_cs/Audi_A8_13/Dynamics_Empty/MuxState ==
  note: mode: Dynamics
  note: mode: Positioning
  note: mode: Dynamics
      | VelVEHICLE
      | wrt VEH
  note: AnglesVEHICLE
      | wrtGLOB
  note: For state mode 'Dynamic' positions
      | are not taken into account, as they
      | are computed by integrating velocity.
      | Click annotation for Help.
  x [m] : Inport  SampleTime=TimeStep
  y [m] : Inport  Port=2  SampleTime=TimeStep
  z [m] : Inport  Port=3  SampleTime=TimeStep
  dx [m/s] : Inport  Port=4  SampleTime=TimeStep
  dy [m/s] : Inport  Port=5  SampleTime=TimeStep
  dz [m/s] : Inport  Port=6  SampleTime=TimeStep
  R [rad] : Inport  Port=7  SampleTime=TimeStep
  P [rad] : Inport  Port=8  SampleTime=TimeStep
  Y [rad] : Inport  Port=9  SampleTime=TimeStep
  Constant : Constant  DisableCoverage=on  Value=positioningmode
  Discrete-Time Integrator : DiscreteIntegrator  SampleTime=TimeStep
  Ground : Ground
  Ground1 : Ground
  Mux1 : Mux  Inputs=[3 3]
  Mux2 : Mux  Inputs=3
  Mux3 : Mux  Inputs=3
  Mux4 : Mux  Inputs=3
  Mux5 : Mux  Inputs=[3 3]
  Mux6 : Mux  Inputs=[6 3]
  Switch : Switch  Threshold=0.5
  Transformation_BODY2GLOBAL : PreScanSimulinkLibrary/Simple_Vehicle_Dynamics/Chassis/MuxDynState/Transformation_BODY2GLOBAL
  mux3 : Mux  Inputs=3
  state : Outport
  wires:
  Constant/1 -> Switch/2
  Mux6/1 -> state/1
  Mux4/1 -> Mux1/1
  Mux5/1 -> Switch/3
  Mux1/1 -> Switch/1
  Switch/1 -> Mux6/1  "PosVeh wrt  GLOB"
  P [rad]/1 -> Mux3/2
  R [rad]/1 -> Mux3/1
  dz [m/s]/1 -> Mux2/3
  dy [m/s]/1 -> Mux2/2
  dx [m/s]/1 -> Mux2/1
  z [m]/1 -> Mux4/3
  y [m]/1 -> Mux4/2
  x [m]/1 -> Mux4/1
  Ground1/1 -> mux3/2  "pitch"
  Y [rad]/1 -> mux3/3, Mux3/3  "yaw"
  Mux3/1 -> Mux6/2
  Transformation_BODY2GLOBAL/1 -> Discrete-Time Integrator/1, Mux5/2  "VelVEH wrt  GLOB"
  mux3/1 -> Transformation_BODY2GLOBAL/2
  Ground/1 -> mux3/1  "roll"
  Mux2/1 -> Mux1/2, Transformation_BODY2GLOBAL/1
  Discrete-Time Integrator/1 -> Mux5/1  "PosVEH wrt  GLOB"

== system ParkAssist_Scenario002_cs/Audi_A8_13/Dynamics_Empty/STATE_Audi_A8_13 ==
  State : Inport  SampleTime=TimeStep
  Bus Creator : BusCreator  Inputs=15  OutDataTypeStr=Bus: PRESCAN_STATEACTUATORDATA  NonVirtualBus=on
  Constant : Constant  Value=0
  Demux : Demux  Outputs=15
  Mux : Mux  Inputs=3
  Mux1 : Mux  Inputs=3
  Mux2 : Mux  Inputs=3
  iniBODYAngles wrtVEH [rad] : Constant  Value=Roll0  SampleTime=TimeStep
  iniBODYAngles wrtVEH [rad]1 : Constant  Value=Pitch0  SampleTime=TimeStep
  iniVEHAngles wrtGLOB [rad] : Constant  Value=Yaw0  SampleTime=TimeStep
  iniVEHposition wrtGLOB [m] : Constant  Value=x0  SampleTime=TimeStep
  iniVEHposition wrtGLOB [m]1 : Constant  Value=y0  SampleTime=TimeStep
  iniVEHposition wrtGLOB [m]2 : Constant  Value=z0  SampleTime=TimeStep
  state2FullState : PreScanSimulinkLibrary/state2FullState  SystemSampleTime=-1
  StateBus : Outport  OutDataTypeStr=Bus: PRESCAN_STATEACTUATORDATA
  wires:
  Mux2/1 -> state2FullState/4
  iniVEHAngles wrtGLOB [rad]/1 -> Mux2/3
  Mux1/1 -> state2FullState/3
  Constant/1 -> Mux2/1, Mux2/2, Mux1/3
  iniBODYAngles wrtVEH [rad]1/1 -> Mux1/2
  iniBODYAngles wrtVEH [rad]/1 -> Mux1/1
  Mux/1 -> state2FullState/2
  iniVEHposition wrtGLOB [m]2/1 -> Mux/3
  iniVEHposition wrtGLOB [m]/1 -> Mux/1
  iniVEHposition wrtGLOB [m]1/1 -> Mux/2
  Demux/15 -> Bus Creator/15  "AngularVelocityYaw"
  Demux/14 -> Bus Creator/14  "AngularVelocityPitch"
  Demux/13 -> Bus Creator/13  "AngularVelocityRoll"
  Demux/12 -> Bus Creator/12  "OrientationYaw"
  Demux/11 -> Bus Creator/11  "OrientationPitch"
  Demux/10 -> Bus Creator/10  "OrientationRoll"
  Demux/9 -> Bus Creator/9  "AccelerationZ"
  Demux/8 -> Bus Creator/8  "AccelerationY"
  Demux/7 -> Bus Creator/7  "AccelerationX"
  Demux/6 -> Bus Creator/6  "VelocityZ"
  Demux/5 -> Bus Creator/5  "VelocityY"
  Demux/4 -> Bus Creator/4  "VelocityX"
  Demux/3 -> Bus Creator/3  "PositionZ"
  Demux/2 -> Bus Creator/2  "PositionY"
  Demux/1 -> Bus Creator/1  "PositionX"
  state2FullState/1 -> Demux/1
  State/1 -> state2FullState/1
  Bus Creator/1 -> StateBus/1

== system ParkAssist_Scenario002_cs/Audi_A8_13/SELF_Demux/compas converter ==
  rotz [rad] : Inport
  cart2compas : Subsystem
  rad2deg : Gain  Gain=180/pi
  heading [deg] : Outport
  wires:
  rad2deg/1 -> cart2compas/1(Angle [deg])
  rotz [rad]/1 -> rad2deg/1
  cart2compas/1(heading [deg]) -> heading [deg]/1

== system ParkAssist_Scenario002_cs/Audi_A8_14/Dynamics_Empty/MuxState ==
  note: mode: Dynamics
  note: mode: Positioning
  note: mode: Dynamics
      | VelVEHICLE
      | wrt VEH
  note: AnglesVEHICLE
      | wrtGLOB
  note: For state mode 'Dynamic' positions
      | are not taken into account, as they
      | are computed by integrating velocity.
      | Click annotation for Help.
  x [m] : Inport  SampleTime=TimeStep
  y [m] : Inport  Port=2  SampleTime=TimeStep
  z [m] : Inport  Port=3  SampleTime=TimeStep
  dx [m/s] : Inport  Port=4  SampleTime=TimeStep
  dy [m/s] : Inport  Port=5  SampleTime=TimeStep
  dz [m/s] : Inport  Port=6  SampleTime=TimeStep
  R [rad] : Inport  Port=7  SampleTime=TimeStep
  P [rad] : Inport  Port=8  SampleTime=TimeStep
  Y [rad] : Inport  Port=9  SampleTime=TimeStep
  Constant : Constant  DisableCoverage=on  Value=positioningmode
  Discrete-Time Integrator : DiscreteIntegrator  SampleTime=TimeStep
  Ground : Ground
  Ground1 : Ground
  Mux1 : Mux  Inputs=[3 3]
  Mux2 : Mux  Inputs=3
  Mux3 : Mux  Inputs=3
  Mux4 : Mux  Inputs=3
  Mux5 : Mux  Inputs=[3 3]
  Mux6 : Mux  Inputs=[6 3]
  Switch : Switch  Threshold=0.5
  Transformation_BODY2GLOBAL : PreScanSimulinkLibrary/Simple_Vehicle_Dynamics/Chassis/MuxDynState/Transformation_BODY2GLOBAL
  mux3 : Mux  Inputs=3
  state : Outport
  wires:
  Constant/1 -> Switch/2
  Mux6/1 -> state/1
  Mux4/1 -> Mux1/1
  Mux5/1 -> Switch/3
  Mux1/1 -> Switch/1
  Switch/1 -> Mux6/1  "PosVeh wrt  GLOB"
  P [rad]/1 -> Mux3/2
  R [rad]/1 -> Mux3/1
  dz [m/s]/1 -> Mux2/3
  dy [m/s]/1 -> Mux2/2
  dx [m/s]/1 -> Mux2/1
  z [m]/1 -> Mux4/3
  y [m]/1 -> Mux4/2
  x [m]/1 -> Mux4/1
  Ground1/1 -> mux3/2  "pitch"
  Y [rad]/1 -> mux3/3, Mux3/3  "yaw"
  Mux3/1 -> Mux6/2
  Transformation_BODY2GLOBAL/1 -> Discrete-Time Integrator/1, Mux5/2  "VelVEH wrt  GLOB"
  mux3/1 -> Transformation_BODY2GLOBAL/2
  Ground/1 -> mux3/1  "roll"
  Mux2/1 -> Mux1/2, Transformation_BODY2GLOBAL/1
  Discrete-Time Integrator/1 -> Mux5/1  "PosVEH wrt  GLOB"

== system ParkAssist_Scenario002_cs/Audi_A8_14/Dynamics_Empty/STATE_Audi_A8_14 ==
  State : Inport  SampleTime=TimeStep
  Bus Creator : BusCreator  Inputs=15  OutDataTypeStr=Bus: PRESCAN_STATEACTUATORDATA  NonVirtualBus=on
  Constant : Constant  Value=0
  Demux : Demux  Outputs=15
  Mux : Mux  Inputs=3
  Mux1 : Mux  Inputs=3
  Mux2 : Mux  Inputs=3
  iniBODYAngles wrtVEH [rad] : Constant  Value=Roll0  SampleTime=TimeStep
  iniBODYAngles wrtVEH [rad]1 : Constant  Value=Pitch0  SampleTime=TimeStep
  iniVEHAngles wrtGLOB [rad] : Constant  Value=Yaw0  SampleTime=TimeStep
  iniVEHposition wrtGLOB [m] : Constant  Value=x0  SampleTime=TimeStep
  iniVEHposition wrtGLOB [m]1 : Constant  Value=y0  SampleTime=TimeStep
  iniVEHposition wrtGLOB [m]2 : Constant  Value=z0  SampleTime=TimeStep
  state2FullState : PreScanSimulinkLibrary/state2FullState  SystemSampleTime=-1
  StateBus : Outport  OutDataTypeStr=Bus: PRESCAN_STATEACTUATORDATA
  wires:
  Mux2/1 -> state2FullState/4
  iniVEHAngles wrtGLOB [rad]/1 -> Mux2/3
  Mux1/1 -> state2FullState/3
  Constant/1 -> Mux2/1, Mux2/2, Mux1/3
  iniBODYAngles wrtVEH [rad]1/1 -> Mux1/2
  iniBODYAngles wrtVEH [rad]/1 -> Mux1/1
  Mux/1 -> state2FullState/2
  iniVEHposition wrtGLOB [m]2/1 -> Mux/3
  iniVEHposition wrtGLOB [m]/1 -> Mux/1
  iniVEHposition wrtGLOB [m]1/1 -> Mux/2
  Demux/15 -> Bus Creator/15  "AngularVelocityYaw"
  Demux/14 -> Bus Creator/14  "AngularVelocityPitch"
  Demux/13 -> Bus Creator/13  "AngularVelocityRoll"
  Demux/12 -> Bus Creator/12  "OrientationYaw"
  Demux/11 -> Bus Creator/11  "OrientationPitch"
  Demux/10 -> Bus Creator/10  "OrientationRoll"
  Demux/9 -> Bus Creator/9  "AccelerationZ"
  Demux/8 -> Bus Creator/8  "AccelerationY"
  Demux/7 -> Bus Creator/7  "AccelerationX"
  Demux/6 -> Bus Creator/6  "VelocityZ"
  Demux/5 -> Bus Creator/5  "VelocityY"
  Demux/4 -> Bus Creator/4  "VelocityX"
  Demux/3 -> Bus Creator/3  "PositionZ"
  Demux/2 -> Bus Creator/2  "PositionY"
  Demux/1 -> Bus Creator/1  "PositionX"
  state2FullState/1 -> Demux/1
  State/1 -> state2FullState/1
  Bus Creator/1 -> StateBus/1

== system ParkAssist_Scenario002_cs/Audi_A8_14/SELF_Demux/compas converter ==
  rotz [rad] : Inport
  cart2compas : Subsystem
  rad2deg : Gain  Gain=180/pi
  heading [deg] : Outport
  wires:
  rad2deg/1 -> cart2compas/1(Angle [deg])
  rotz [rad]/1 -> rad2deg/1
  cart2compas/1(heading [deg]) -> heading [deg]/1

== system ParkAssist_Scenario002_cs/Audi_A8_2/Dynamics_Empty/MuxState ==
  note: mode: Dynamics
  note: mode: Positioning
  note: mode: Dynamics
      | VelVEHICLE
      | wrt VEH
  note: AnglesVEHICLE
      | wrtGLOB
  note: For state mode 'Dynamic' positions
      | are not taken into account, as they
      | are computed by integrating velocity.
      | Click annotation for Help.
  x [m] : Inport  SampleTime=TimeStep
  y [m] : Inport  Port=2  SampleTime=TimeStep
  z [m] : Inport  Port=3  SampleTime=TimeStep
  dx [m/s] : Inport  Port=4  SampleTime=TimeStep
  dy [m/s] : Inport  Port=5  SampleTime=TimeStep
  dz [m/s] : Inport  Port=6  SampleTime=TimeStep
  R [rad] : Inport  Port=7  SampleTime=TimeStep
  P [rad] : Inport  Port=8  SampleTime=TimeStep
  Y [rad] : Inport  Port=9  SampleTime=TimeStep
  Constant : Constant  DisableCoverage=on  Value=positioningmode
  Discrete-Time Integrator : DiscreteIntegrator  SampleTime=TimeStep
  Ground : Ground
  Ground1 : Ground
  Mux1 : Mux  Inputs=[3 3]
  Mux2 : Mux  Inputs=3
  Mux3 : Mux  Inputs=3
  Mux4 : Mux  Inputs=3
  Mux5 : Mux  Inputs=[3 3]
  Mux6 : Mux  Inputs=[6 3]
  Switch : Switch  Threshold=0.5
  Transformation_BODY2GLOBAL : PreScanSimulinkLibrary/Simple_Vehicle_Dynamics/Chassis/MuxDynState/Transformation_BODY2GLOBAL
  mux3 : Mux  Inputs=3
  state : Outport
  wires:
  Constant/1 -> Switch/2
  Mux6/1 -> state/1
  Mux4/1 -> Mux1/1
  Mux5/1 -> Switch/3
  Mux1/1 -> Switch/1
  Switch/1 -> Mux6/1  "PosVeh wrt  GLOB"
  P [rad]/1 -> Mux3/2
  R [rad]/1 -> Mux3/1
  dz [m/s]/1 -> Mux2/3
  dy [m/s]/1 -> Mux2/2
  dx [m/s]/1 -> Mux2/1
  z [m]/1 -> Mux4/3
  y [m]/1 -> Mux4/2
  x [m]/1 -> Mux4/1
  Ground1/1 -> mux3/2  "pitch"
  Y [rad]/1 -> mux3/3, Mux3/3  "yaw"
  Mux3/1 -> Mux6/2
  Transformation_BODY2GLOBAL/1 -> Discrete-Time Integrator/1, Mux5/2  "VelVEH wrt  GLOB"
  mux3/1 -> Transformation_BODY2GLOBAL/2
  Ground/1 -> mux3/1  "roll"
  Mux2/1 -> Mux1/2, Transformation_BODY2GLOBAL/1
  Discrete-Time Integrator/1 -> Mux5/1  "PosVEH wrt  GLOB"

== system ParkAssist_Scenario002_cs/Audi_A8_2/Dynamics_Empty/STATE_Audi_A8_2 ==
  State : Inport  SampleTime=TimeStep
  Bus Creator : BusCreator  Inputs=15  OutDataTypeStr=Bus: PRESCAN_STATEACTUATORDATA  NonVirtualBus=on
  Constant : Constant  Value=0
  Demux : Demux  Outputs=15
  Mux : Mux  Inputs=3
  Mux1 : Mux  Inputs=3
  Mux2 : Mux  Inputs=3
  iniBODYAngles wrtVEH [rad] : Constant  Value=Roll0  SampleTime=TimeStep
  iniBODYAngles wrtVEH [rad]1 : Constant  Value=Pitch0  SampleTime=TimeStep
  iniVEHAngles wrtGLOB [rad] : Constant  Value=Yaw0  SampleTime=TimeStep
  iniVEHposition wrtGLOB [m] : Constant  Value=x0  SampleTime=TimeStep
  iniVEHposition wrtGLOB [m]1 : Constant  Value=y0  SampleTime=TimeStep
  iniVEHposition wrtGLOB [m]2 : Constant  Value=z0  SampleTime=TimeStep
  state2FullState : PreScanSimulinkLibrary/state2FullState  SystemSampleTime=-1
  StateBus : Outport  OutDataTypeStr=Bus: PRESCAN_STATEACTUATORDATA
  wires:
  Mux2/1 -> state2FullState/4
  iniVEHAngles wrtGLOB [rad]/1 -> Mux2/3
  Mux1/1 -> state2FullState/3
  Constant/1 -> Mux2/1, Mux2/2, Mux1/3
  iniBODYAngles wrtVEH [rad]1/1 -> Mux1/2
  iniBODYAngles wrtVEH [rad]/1 -> Mux1/1
  Mux/1 -> state2FullState/2
  iniVEHposition wrtGLOB [m]2/1 -> Mux/3
  iniVEHposition wrtGLOB [m]/1 -> Mux/1
  iniVEHposition wrtGLOB [m]1/1 -> Mux/2
  Demux/15 -> Bus Creator/15  "AngularVelocityYaw"
  Demux/14 -> Bus Creator/14  "AngularVelocityPitch"
  Demux/13 -> Bus Creator/13  "AngularVelocityRoll"
  Demux/12 -> Bus Creator/12  "OrientationYaw"
  Demux/11 -> Bus Creator/11  "OrientationPitch"
  Demux/10 -> Bus Creator/10  "OrientationRoll"
  Demux/9 -> Bus Creator/9  "AccelerationZ"
  Demux/8 -> Bus Creator/8  "AccelerationY"
  Demux/7 -> Bus Creator/7  "AccelerationX"
  Demux/6 -> Bus Creator/6  "VelocityZ"
  Demux/5 -> Bus Creator/5  "VelocityY"
  Demux/4 -> Bus Creator/4  "VelocityX"
  Demux/3 -> Bus Creator/3  "PositionZ"
  Demux/2 -> Bus Creator/2  "PositionY"
  Demux/1 -> Bus Creator/1  "PositionX"
  state2FullState/1 -> Demux/1
  State/1 -> state2FullState/1
  Bus Creator/1 -> StateBus/1

== system ParkAssist_Scenario002_cs/Audi_A8_2/SELF_Demux/compas converter ==
  rotz [rad] : Inport
  cart2compas : Subsystem
  rad2deg : Gain  Gain=180/pi
  heading [deg] : Outport
  wires:
  rad2deg/1 -> cart2compas/1(Angle [deg])
  rotz [rad]/1 -> rad2deg/1
  cart2compas/1(heading [deg]) -> heading [deg]/1

== system ParkAssist_Scenario002_cs/Audi_A8_3/Dynamics_Empty/MuxState ==
  note: mode: Dynamics
  note: mode: Positioning
  note: mode: Dynamics
      | VelVEHICLE
      | wrt VEH
  note: AnglesVEHICLE
      | wrtGLOB
  note: For state mode 'Dynamic' positions
      | are not taken into account, as they
      | are computed by integrating velocity.
      | Click annotation for Help.
  x [m] : Inport  SampleTime=TimeStep
  y [m] : Inport  Port=2  SampleTime=TimeStep
  z [m] : Inport  Port=3  SampleTime=TimeStep
  dx [m/s] : Inport  Port=4  SampleTime=TimeStep
  dy [m/s] : Inport  Port=5  SampleTime=TimeStep
  dz [m/s] : Inport  Port=6  SampleTime=TimeStep
  R [rad] : Inport  Port=7  SampleTime=TimeStep
  P [rad] : Inport  Port=8  SampleTime=TimeStep
  Y [rad] : Inport  Port=9  SampleTime=TimeStep
  Constant : Constant  DisableCoverage=on  Value=positioningmode
  Discrete-Time Integrator : DiscreteIntegrator  SampleTime=TimeStep
  Ground : Ground
  Ground1 : Ground
  Mux1 : Mux  Inputs=[3 3]
  Mux2 : Mux  Inputs=3
  Mux3 : Mux  Inputs=3
  Mux4 : Mux  Inputs=3
  Mux5 : Mux  Inputs=[3 3]
  Mux6 : Mux  Inputs=[6 3]
  Switch : Switch  Threshold=0.5
  Transformation_BODY2GLOBAL : PreScanSimulinkLibrary/Simple_Vehicle_Dynamics/Chassis/MuxDynState/Transformation_BODY2GLOBAL
  mux3 : Mux  Inputs=3
  state : Outport
  wires:
  Constant/1 -> Switch/2
  Mux6/1 -> state/1
  Mux4/1 -> Mux1/1
  Mux5/1 -> Switch/3
  Mux1/1 -> Switch/1
  Switch/1 -> Mux6/1  "PosVeh wrt  GLOB"
  P [rad]/1 -> Mux3/2
  R [rad]/1 -> Mux3/1
  dz [m/s]/1 -> Mux2/3
  dy [m/s]/1 -> Mux2/2
  dx [m/s]/1 -> Mux2/1
  z [m]/1 -> Mux4/3
  y [m]/1 -> Mux4/2
  x [m]/1 -> Mux4/1
  Ground1/1 -> mux3/2  "pitch"
  Y [rad]/1 -> mux3/3, Mux3/3  "yaw"
  Mux3/1 -> Mux6/2
  Transformation_BODY2GLOBAL/1 -> Discrete-Time Integrator/1, Mux5/2  "VelVEH wrt  GLOB"
  mux3/1 -> Transformation_BODY2GLOBAL/2
  Ground/1 -> mux3/1  "roll"
  Mux2/1 -> Mux1/2, Transformation_BODY2GLOBAL/1
  Discrete-Time Integrator/1 -> Mux5/1  "PosVEH wrt  GLOB"

== system ParkAssist_Scenario002_cs/Audi_A8_3/Dynamics_Empty/STATE_Audi_A8_3 ==
  State : Inport  SampleTime=TimeStep
  Bus Creator : BusCreator  Inputs=15  OutDataTypeStr=Bus: PRESCAN_STATEACTUATORDATA  NonVirtualBus=on
  Constant : Constant  Value=0
  Demux : Demux  Outputs=15
  Mux : Mux  Inputs=3
  Mux1 : Mux  Inputs=3
  Mux2 : Mux  Inputs=3
  iniBODYAngles wrtVEH [rad] : Constant  Value=Roll0  SampleTime=TimeStep
  iniBODYAngles wrtVEH [rad]1 : Constant  Value=Pitch0  SampleTime=TimeStep
  iniVEHAngles wrtGLOB [rad] : Constant  Value=Yaw0  SampleTime=TimeStep
  iniVEHposition wrtGLOB [m] : Constant  Value=x0  SampleTime=TimeStep
  iniVEHposition wrtGLOB [m]1 : Constant  Value=y0  SampleTime=TimeStep
  iniVEHposition wrtGLOB [m]2 : Constant  Value=z0  SampleTime=TimeStep
  state2FullState : PreScanSimulinkLibrary/state2FullState  SystemSampleTime=-1
  StateBus : Outport  OutDataTypeStr=Bus: PRESCAN_STATEACTUATORDATA
  wires:
  Mux2/1 -> state2FullState/4
  iniVEHAngles wrtGLOB [rad]/1 -> Mux2/3
  Mux1/1 -> state2FullState/3
  Constant/1 -> Mux2/1, Mux2/2, Mux1/3
  iniBODYAngles wrtVEH [rad]1/1 -> Mux1/2
  iniBODYAngles wrtVEH [rad]/1 -> Mux1/1
  Mux/1 -> state2FullState/2
  iniVEHposition wrtGLOB [m]2/1 -> Mux/3
  iniVEHposition wrtGLOB [m]/1 -> Mux/1
  iniVEHposition wrtGLOB [m]1/1 -> Mux/2
  Demux/15 -> Bus Creator/15  "AngularVelocityYaw"
  Demux/14 -> Bus Creator/14  "AngularVelocityPitch"
  Demux/13 -> Bus Creator/13  "AngularVelocityRoll"
  Demux/12 -> Bus Creator/12  "OrientationYaw"
  Demux/11 -> Bus Creator/11  "OrientationPitch"
  Demux/10 -> Bus Creator/10  "OrientationRoll"
  Demux/9 -> Bus Creator/9  "AccelerationZ"
  Demux/8 -> Bus Creator/8  "AccelerationY"
  Demux/7 -> Bus Creator/7  "AccelerationX"
  Demux/6 -> Bus Creator/6  "VelocityZ"
  Demux/5 -> Bus Creator/5  "VelocityY"
  Demux/4 -> Bus Creator/4  "VelocityX"
  Demux/3 -> Bus Creator/3  "PositionZ"
  Demux/2 -> Bus Creator/2  "PositionY"
  Demux/1 -> Bus Creator/1  "PositionX"
  state2FullState/1 -> Demux/1
  State/1 -> state2FullState/1
  Bus Creator/1 -> StateBus/1

== system ParkAssist_Scenario002_cs/Audi_A8_3/SELF_Demux/compas converter ==
  rotz [rad] : Inport
  cart2compas : Subsystem
  rad2deg : Gain  Gain=180/pi
  heading [deg] : Outport
  wires:
  rad2deg/1 -> cart2compas/1(Angle [deg])
  rotz [rad]/1 -> rad2deg/1
  cart2compas/1(heading [deg]) -> heading [deg]/1
